simulink model "diagram_simulink"  (R2023b)
settings: Solver=VariableStepAuto  StartTime=0.0  StopTime=200  RelTol=1e-3
model workspace (MAT data in the model file):
  kp2 = 1
libraries: cstblocks x4
settings Model: Creator=boliy  LastModifiedBy=Admin

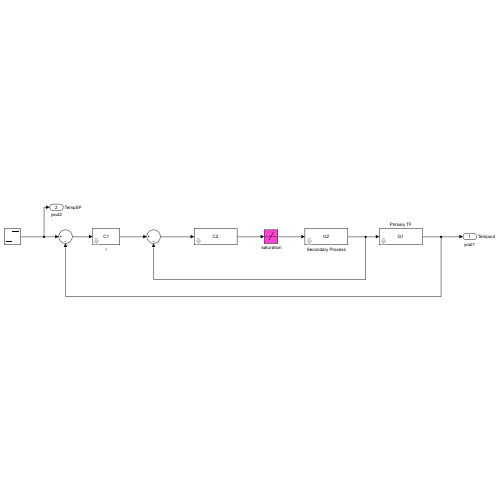
[thumbnail: Simulink's stored preview of the top-level diagram]
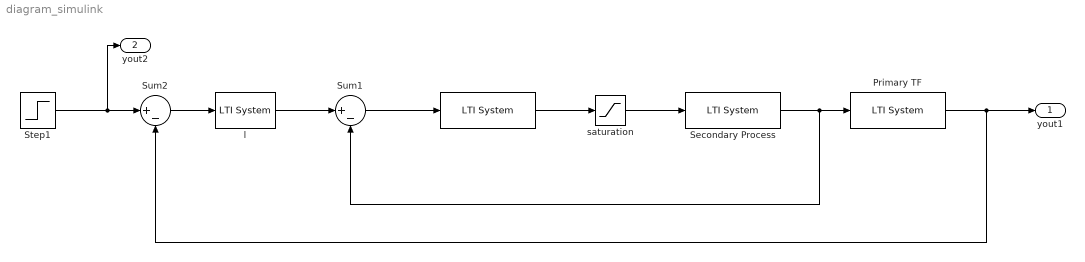
== system diagram_simulink ==
  " " : cstblocks/LTI System  sys=C2  IC=[]  PadeOrder=0
  " saturation" : Saturate  UpperLimit=1  LowerLimit=-1
  Primary TF : cstblocks/LTI System  sys=G1  IC=[]  PadeOrder=0
  Secondary Process : cstblocks/LTI System  sys=G2  IC=[]  PadeOrder=0
  Step1 : Step  Time=0  SampleTime=0.1
  Sum1 : Sum  Inputs=|+-
  Sum2 : Sum  Inputs=|+-
  l : cstblocks/LTI System  sys=C1  IC=[]  PadeOrder=0
  yout1 : Outport  SignalName=Tempout  VectorParamsAs1DForOutWhenUnconnected=off
  yout2 : Outport  Port=2  SignalName=TempSP  VectorParamsAs1DForOutWhenUnconnected=off
  wires:
  " "/1 -> " saturation"/1
  Sum1/1 -> " "/1
  Secondary Process/1 -> Primary TF/1, Sum1/2
  l/1 -> Sum1/1
  Primary TF/1 -> yout1/1, Sum2/2
  Step1/1 -> Sum2/1, yout2/1
  Sum2/1 -> l/1
  " saturation"/1 -> Secondary Process/1
